simulink model "VDCHyd2022a"  (R2022a)
settings: Solver=daessc  StartTime=0.0  StopTime=simulationEndTime  FixedStep=0.001  RelTol=1e-2
values from neighbouring files (symbols this model uses):
  aux = thetaXrLB(i)    [initInertiaUpdate.m]
  Bc1_V = [0;0;0;0;0;0]    [InitializeSimulationParameters.m]
  Bc1_Vr = [0;0;0;0;0;0]    [InitializeSimulationParameters.m]
  D22Fr = [0;0;0;0;0;0]    [InitializeSimulationParameters.m]
  filtDF = init2ndOrderLowPassFilter(filtDF.cutOffFrequency,1,controller.dT)    [initializeLowPassFilters.m]
  filtDV = init2ndOrderLowPassFilter(filtDV.cutOffFrequency,1,controller.dT)    [initializeLowPassFilters.m]
  filtEnc = init2ndOrderLowPassFilter(filtEnc.cutOffFrequency,1,controller.dT)    [initializeLowPassFilters.m]
  filtPres = init2ndOrderLowPassFilter(filtPres.cutOffFrequency,1,controller.dT)    [initializeLowPassFilters.m]
  MODE = 1    [RUN_ME.m]
  s = tf('s')    [init2ndOrderLowPassFilter.m]
undefined symbols (not defined in the file or in its folder): B11_r_B11Tc1, B11_V, B11_Vr, B11Ftot_r, B12_r_B12Tc2, B12_Rot_Tc2, B12_U_Tc2, B12_V, B12_Vr, B12Ftot_r, B31_r_B31B41, B31_V, B31_Vr, B31FTot_r, B32_r_B32B42, B32_Rot_B42, B32_U_B42, B32_V, B32_Vr, B32FTot_r, B41_r_B41Tc1, B41_V, B41_Vr, B41FTot_r, B42_r_B42Tc2, B42_Rot_Tc2, B42_U_Tc2, B42_V, B42_Vr, B42FTot_r, B52_r_B52P32, B52_Rot_P32, B52_U_P32, B52_V, B52_Vr, B52Ftot_r, Bc1_r_Bc1B11, Bc1_r_Bc1B31, Bc1FTot_r, Bc2_r_Bc2B12, Bc2_r_Bc2B32, Bc2_Rot_B12, Bc2_Rot_B32, Bc2_U_B12, Bc2_U_B32, Bc2_V, Bc2_Vr, Bc2Tot_r, controller, cyl1, cyl2, cylT2, D22_V, D22_Vr, DiscIntNeverNeededParam, dq1, dq11, dq11r, dq12, dq12r ... (+119)
libraries: sm_lib x34, nesl_utility x15, simulink x11, dspinverses x1
(part 12 of 12)

== matlab function VDCHyd2022a/sbVDCController/sbFormTotalRequiredForces/sbTotalRequiredForcesRS1/regressorYB41r ==
  data: B41Vr input; B41dVr input; B41V input; B41_Rot_W input; gravity parameter; YB41r output
function YB41r  = inertiaRegressor(B41Vr, B41dVr, B41V, B41_Rot_W,  gravity)

    % Forms regressor matrix YB41r as described in Appendix A of
    % Zhu, Wen-Hong. Virtual decomposition control: toward hyper degrees
    % of freedom robots. Vol. 60. Springer Science & Business Media, 2010.

    % The code below is not the most apparent 1-to-1 visual mapping to the
    % book equations since it was generated using a symbolic toolbox.
    
    vxr = B41Vr(1); vyr = B41Vr(2); vzr = B41Vr(3);
    wxr = B41Vr(4); wyr = B41Vr(5); wzr = B41Vr(6);
    
    axr = B41dVr(1); ayr = B41dVr(2); azr = B41dVr(3);
    dwxr = B41dVr(4); dwyr = B41dVr(5); dwzr = B41dVr(6);
    
    wx = B41V(4); wy = B41V(5); wz = B41V(6);
    
    B41g = B41_Rot_W*gravity.Wg;
    
    gx = B41g(1);
    gy = B41g(2);
    gz = B41g(3);
    
    Y11 = (-vyr * wz + vzr * wy + axr + gx);
    t5 = (wy * wyr);
    t6 = (wz * wzr);
    Y12 = -t5 - t6;
    t7 = (wxr * wy);
    Y13 = (t7 - dwzr);
    t8 = (wxr * wz);
    Y14  = (t8 + dwyr);
    Y15 = 0;
    Y16 = 0;
    Y17 = 0;
    Y18  = 0;
    Y19 = 0;
    Y110 = 0;
    Y111 = 0;
    Y112 = 0;
    Y113 = 0;
    Y21 = vxr * wz - vzr * wx + ayr + gy;
    t11 = wx * wyr;
    Y22 = t11 + dwzr;
    t12 = wx * wxr;
    Y23 = -t12 - t6;
    t13 = wyr * wz;
    Y24 = t13 - dwxr;
    Y25 = 0;
    Y26 = 0;
    Y27 = 0;
    Y28 = 0;
    Y29 = 0;
    Y210 = 0;
    Y211 = 0;
    Y212 = 0;
    Y213 = 0;
    Y31 = -vxr * wy + vyr * wx + azr + gz;
    t16 = wx * wzr;
    Y32 = t16 - dwyr;
    t17 = wy * wzr;
    Y33 = t17 + dwxr;
    Y34 = -t12 - t5;
    Y35 = 0;
    Y36 = 0;
    Y37 = 0;
    Y38 = 0;
    Y39 = 0;
    Y310 = 0;
    Y311 = 0;
    Y312 = 0;
    Y313 = 0;
    Y41 = 0;
    Y42 = 0;
    Y43 = Y31;
    Y44 = -Y21;
    Y45 = 0;
    Y46 = Y33;
    Y47 = -Y24;
    Y48 = Y32;
    Y49 = -Y22;
    Y410 = -t5 + t6;
    Y411 = t17 - t13 + dwxr;
    Y412 = -t13;
    Y413 = t17;
    Y51 = 0;
    Y52 = -Y43;
    Y53 = 0;
    Y54 = Y11;
    Y55 = -Y48;
    Y56 = 0;
    Y57 = Y14;
    Y58 = -Y46;
    Y59 = t12 - t6;
    Y510 = Y13;
    Y511 = t8;
    Y512 = -t16 + Y511 + dwyr;
    Y513 = -t16;
    Y61 = 0;
    Y62 = Y21;
    Y63 = -Y54;
    Y64 = 0;
    Y65 = Y22;
    Y66 = -Y510;
    Y67 = 0;
    Y68 = -t12 + t5;
    Y69 = Y24;
    Y610 = -Y57;
    Y611 = -t7;
    Y612 = t11;
    Y613 = Y612 + Y611 + dwzr;
    
    
    YB41r = [Y11 Y12 Y13 Y14 Y15 Y16 Y17 Y18 Y19 Y110 Y111 Y112 Y113;...
             Y21 Y22 Y23 Y24 Y25 Y26 Y27 Y28 Y29 Y210 Y211 Y212 Y213;...
             Y31 Y32 Y33 Y34 Y35 Y36 Y37 Y38 Y39 Y310 Y311 Y312 Y313;...
             Y41 Y42 Y43 Y44 Y45 Y46 Y47 Y48 Y49 Y410 Y411 Y412 Y413;...
             Y51 Y52 Y53 Y54 Y55 Y56 Y57 Y58 Y59 Y510 Y511 Y512 Y513;...
             Y61 Y62 Y63 Y64 Y65 Y66 Y67 Y68 Y69 Y610 Y611 Y612 Y613];

end

== matlab function VDCHyd2022a/sbVDCController/sbFormTotalRequiredForces/sbTotalRequiredForcesRS1/regressorYBc1r ==
  data: Bc1Vr input; Bc1dVr input; Bc1V input; Bc1_Rot_W input; gravity parameter; YBc1r output
function YBc1r  = inertiaRegressor(Bc1Vr, Bc1dVr, Bc1V, Bc1_Rot_W,  gravity)

    % Forms regressor matrix YBc1r as described in Appendix A of
    % Zhu, Wen-Hong. Virtual decomposition control: toward hyper degrees
    % of freedom robots. Vol. 60. Springer Science & Business Media, 2010.

    % The code below is not the most apparent 1-to-1 visual mapping to the
    % book equations since it was generated using a symbolic toolbox.

    vxr = Bc1Vr(1); vyr = Bc1Vr(2); vzr = Bc1Vr(3);
    wxr = Bc1Vr(4); wyr = Bc1Vr(5); wzr = Bc1Vr(6);
    
    axr = Bc1dVr(1); ayr = Bc1dVr(2); azr = Bc1dVr(3);
    dwxr = Bc1dVr(4); dwyr = Bc1dVr(5); dwzr = Bc1dVr(6);
    
    wx = Bc1V(4); wy = Bc1V(5); wz = Bc1V(6);
    
    Bc1g = Bc1_Rot_W*gravity.Wg;
    
    gx = Bc1g(1); gy = Bc1g(2); gz = Bc1g(3);
    
    Y11 = (-vyr * wz + vzr * wy + axr + gx);
    t5 = (wy * wyr);
    t6 = (wz * wzr);
    Y12 = -t5 - t6;
    t7 = (wxr * wy);
    Y13 = (t7 - dwzr);
    t8 = (wxr * wz);
    Y14  = (t8 + dwyr);
    Y15 = 0;
    Y16 = 0;
    Y17 = 0;
    Y18  = 0;
    Y19 = 0;
    Y110 = 0;
    Y111 = 0;
    Y112 = 0;
    Y113 = 0;
    Y21 = vxr * wz - vzr * wx + ayr + gy;
    t11 = wx * wyr;
    Y22 = t11 + dwzr;
    t12 = wx * wxr;
    Y23 = -t12 - t6;
    t13 = wyr * wz;
    Y24 = t13 - dwxr;
    Y25 = 0;
    Y26 = 0;
    Y27 = 0;
    Y28 = 0;
    Y29 = 0;
    Y210 = 0;
    Y211 = 0;
    Y212 = 0;
    Y213 = 0;
    Y31 = -vxr * wy + vyr * wx + azr + gz;
    t16 = wx * wzr;
    Y32 = t16 - dwyr;
    t17 = wy * wzr;
    Y33 = t17 + dwxr;
    Y34 = -t12 - t5;
    Y35 = 0;
    Y36 = 0;
    Y37 = 0;
    Y38 = 0;
    Y39 = 0;
    Y310 = 0;
    Y311 = 0;
    Y312 = 0;
    Y313 = 0;
    Y41 = 0;
    Y42 = 0;
    Y43 = Y31;
    Y44 = -Y21;
    Y45 = 0;
    Y46 = Y33;
    Y47 = -Y24;
    Y48 = Y32;
    Y49 = -Y22;
    Y410 = -t5 + t6;
    Y411 = t17 - t13 + dwxr;
    Y412 = -t13;
    Y413 = t17;
    Y51 = 0;
    Y52 = -Y43;
    Y53 = 0;
    Y54 = Y11;
    Y55 = -Y48;
    Y56 = 0;
    Y57 = Y14;
    Y58 = -Y46;
    Y59 = t12 - t6;
    Y510 = Y13;
    Y511 = t8;
    Y512 = -t16 + Y511 + dwyr;
    Y513 = -t16;
    Y61 = 0;
    Y62 = Y21;
    Y63 = -Y54;
    Y64 = 0;
    Y65 = Y22;
    Y66 = -Y510;
    Y67 = 0;
    Y68 = -t12 + t5;
    Y69 = Y24;
    Y610 = -Y57;
    Y611 = -t7;
    Y612 = t11;
    Y613 = Y612 + Y611 + dwzr;
    
    
    YBc1r = [Y11 Y12 Y13 Y14 Y15 Y16 Y17 Y18 Y19 Y110 Y111 Y112 Y113;...
             Y21 Y22 Y23 Y24 Y25 Y26 Y27 Y28 Y29 Y210 Y211 Y212 Y213;...
             Y31 Y32 Y33 Y34 Y35 Y36 Y37 Y38 Y39 Y310 Y311 Y312 Y313;...
             Y41 Y42 Y43 Y44 Y45 Y46 Y47 Y48 Y49 Y410 Y411 Y412 Y413;...
             Y51 Y52 Y53 Y54 Y55 Y56 Y57 Y58 Y59 Y510 Y511 Y512 Y513;...
             Y61 Y62 Y63 Y64 Y65 Y66 Y67 Y68 Y69 Y610 Y611 Y612 Y613];

end

== matlab function VDCHyd2022a/sbVDCController/sbFormingControlActions/controlVoltageRS1 ==
  data: uf1r input; pS input; pR input; pa1 input; pb1 input; x1 input; thetav1 input; u1 output; hosing1 parameter; cyl1 parameter
function u1  = calculateControlVoltage(uf1r, pS, pR, pa1, pb1, x1, thetav1, hosing1, cyl1)

    cp1 = thetav1(1); cn1=thetav1(2); cp2=thetav1(3); cn2=thetav1(4);

    % Implemented per (27) in S. Lampinen, J. Koivumäki and J. Mattila, 
    % "Improved Hydraulic Cylinder Model for the Virtual Decomposition 
    % Control Approach," 2019 IEEE International Conference on Cybernetics 
    % and Intelligent Systems (CIS) and IEEE Conference on Robotics, 
    % Automation and Mechatronics (RAM), Bangkok, Thailand, 2019, 
    % pp. 113-118, doi: 10.1109/CIS-RAM47153.2019.9095788 
    u1 = uf1r*selFcn(uf1r)/( (cp1*sqAbsPresDrop(pS-pa1))/(hosing1.V0a/cyl1.Aa + x1) + (cn2*sqAbsPresDrop(pb1-pR))/(hosing1.V0b/cyl1.Ab + cyl1.sp - x1) ) + ...
         uf1r*selFcn(-uf1r)/( (cp2*sqAbsPresDrop(pS-pb1))/(hosing1.V0b/cyl1.Ab + cyl1.sp - x1) + (cn1*sqAbsPresDrop(pa1-pR))/(hosing1.V0a/cyl1.Aa + x1) );


end


function S = selFcn(U)

    if U > 0
        S = 1;
    else
        S = 0;
    end
    
end

function nup = sqAbsPresDrop(dp)

    nup = sign(dp)*sqrt(abs(dp));

end

== matlab function VDCHyd2022a/sbVDCController/sbFormingControlActions/regressorYd1 ==
  data: dfp1r input; Yd1 output; x1 input; dx1 input; pa1 input; pb1 input; hosing1 parameter; cyl1 parameter
function Yd1 = cylinderRegressor(dfp1r, x1, dx1, pa1, pb1, hosing1, cyl1)

    % Implemented per (43) in S. Lampinen, J. Koivumäki and J. Mattila, 
    % "Improved Hydraulic Cylinder Model for the Virtual Decomposition 
    % Control Approach," 2019 IEEE International Conference on Cybernetics 
    % and Intelligent Systems (CIS) and IEEE Conference on Robotics, 
    % Automation and Mechatronics (RAM), Bangkok, Thailand, 2019, 
    % pp. 113-118, doi: 10.1109/CIS-RAM47153.2019.9095788.
    Yd1 = [dfp1r,...
           dx1/(hosing1.V0a/cyl1.Aa + x1),...
           dx1/(hosing1.V0b/cyl1.Ab + cyl1.sp - x1),...
           ((pa1-pb1)*(cyl1.Aa*hosing1.V0b + cyl1.Ab*hosing1.V0a + cyl1.Aa*cyl1.Ab*cyl1.sp))/((hosing1.V0a + cyl1.Aa*x1)*(hosing1.V0b + cyl1.Ab*(cyl1.sp - x1)))];

end

== matlab function VDCHyd2022a/sbVDCController/sbFormingControlActions/regressorYvt2 ==
  data: ut2 input; Yvt2 output; pS input; pR input; pat2 input; pbt2 input; xt2 input; hosingT2 parameter; cylT2 parameter
function Yvt2 = valveRegressor(ut2, pS, pR, pat2, pbt2, xt2, hosingT2, cylT2)

    % Implemented per (25) in S. Lampinen, J. Koivumäki and J. Mattila, 
    % "Improved Hydraulic Cylinder Model for the Virtual Decomposition 
    % Control Approach," 2019 IEEE International Conference on Cybernetics 
    % and Intelligent Systems (CIS) and IEEE Conference on Robotics, 
    % Automation and Mechatronics (RAM), Bangkok, Thailand, 2019, 
    % pp. 113-118, doi: 10.1109/CIS-RAM47153.2019.9095788 in order
    % Yv = [cp1, cn1, cp2, cn2]
    Yvt2 = [sqAbsPresDrop(pS - pat2)*selFcn(ut2)*ut2/(hosingT2.V0a/cylT2.Aa + xt2),...
            sqAbsPresDrop(pat2 - pR)*selFcn(-ut2)*ut2/(hosingT2.V0a/cylT2.Aa + xt2),...
            sqAbsPresDrop(pS - pbt2)*selFcn(-ut2)*ut2/(hosingT2.V0b/cylT2.Ab + cylT2.sp - xt2),...
            sqAbsPresDrop(pbt2 - pR)*selFcn(ut2)*ut2/(hosingT2.V0b/cylT2.Ab + cylT2.sp - xt2)];

end

function S = selFcn(U)

    if U > 0
        S = 1;
    else
        S = 0;
    end
    
end

function nup = sqAbsPresDrop(dp)

    nup = sign(dp)*sqrt(abs(dp));

end

== matlab function VDCHyd2022a/sbVDCController/sbFormingControlActions/regressorYd2 ==
  data: dfp2r input; Yd2 output; x2 input; dx2 input; pa2 input; pb2 input; hosing2 parameter; cyl2 parameter
function Yd2 = cylinderRegressor(dfp2r, x2, dx2, pa2, pb2, hosing2, cyl2)
    
    % Implemented per (43) in S. Lampinen, J. Koivumäki and J. Mattila, 
    % "Improved Hydraulic Cylinder Model for the Virtual Decomposition 
    % Control Approach," 2019 IEEE International Conference on Cybernetics 
    % and Intelligent Systems (CIS) and IEEE Conference on Robotics, 
    % Automation and Mechatronics (RAM), Bangkok, Thailand, 2019, 
    % pp. 113-118, doi: 10.1109/CIS-RAM47153.2019.9095788.
    Yd2 = [dfp2r,...
           dx2/(hosing2.V0a/cyl2.Aa + x2),...
           dx2/(hosing2.V0b/cyl2.Ab + cyl2.sp - x2),...
           ((pa2-pb2)*(cyl2.Aa*hosing2.V0b + cyl2.Ab*hosing2.V0a + cyl2.Aa*cyl2.Ab*cyl2.sp))/((hosing2.V0a + cyl2.Aa*x2)*(hosing2.V0b + cyl2.Ab*(cyl2.sp - x2)))];

end
